simulink subsystem "SCIOutAbstractionOpenLoop"  (R2024b)
settings: Solver=VariableStepAuto  StartTime=0.0  StopTime=10.0  RelTol=1e-3
libraries: svdutilitieslib x1
settings Model: Creator=The MathWorks, Inc.  LastModifiedBy=snarayan
settings RTWCC: GPUComputeCapability=3.5  LargeConstantGeneration=WriteOnlyDNNConstantsToDataFiles

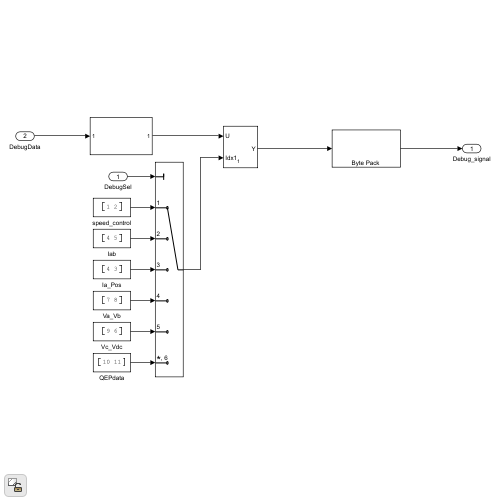
[thumbnail: Simulink's stored preview of the top-level diagram]
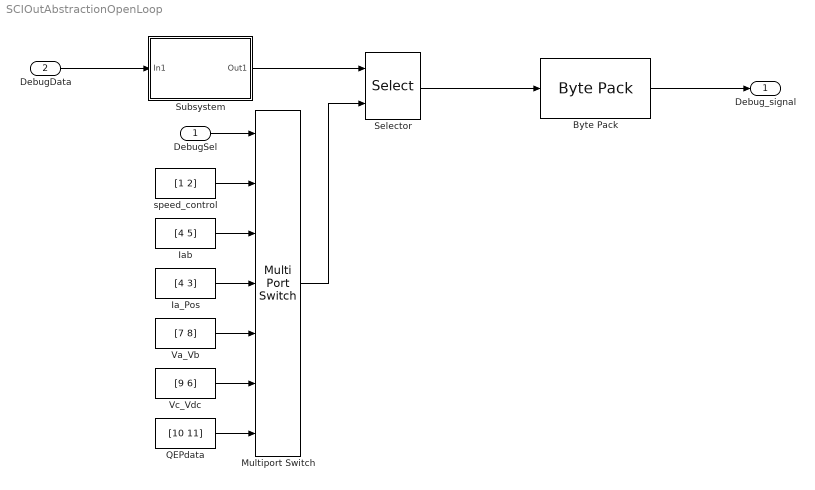
== system SCIOutAbstractionOpenLoop ==
  DebugSel : Inport
  DebugData : Inport  Port=2
  Byte Pack : svdutilitieslib/Byte Pack  maskPackedDataType=uint8  datatypes={'single'}  byteAlign=1  blockPlatform=tic2000
  Ia_Pos : Constant  Value=[4 3]  OutDataTypeStr=uint16  SampleTime=-1
  Iab : Constant  Value=[4 5]  OutDataTypeStr=uint16  SampleTime=-1
  Multiport Switch : MultiPortSwitch  Inputs=6  DiagnosticForDefault=Warning  OutDataTypeStr=uint16  RndMeth=Simplest  SaturateOnIntegerOverflow=off  InputSameDT=off
  QEPdata : Constant  Value=[10 11]  OutDataTypeStr=uint16  SampleTime=-1
  Selector : Selector  InputPortWidth=11  IndexOptions=Index vector (port)  Indices=[1 3]  OutputSizes=1
  Subsystem : Subsystem
  Va_Vb : Constant  Value=[7 8]  OutDataTypeStr=uint16  SampleTime=-1
  Vc_Vdc : Constant  Value=[9 6]  OutDataTypeStr=uint16  SampleTime=-1
  speed_control : Constant  Value=[1 2]  OutDataTypeStr=uint16  SampleTime=-1
  Debug_signal : Outport
  wires:
  speed_control/1 -> Multiport Switch/2
  Multiport Switch/1 -> Selector/2
  DebugSel/1 -> Multiport Switch/1
  Selector/1 -> Byte Pack/1
  Byte Pack/1 -> Debug_signal/1
  Iab/1 -> Multiport Switch/3
  Ia_Pos/1 -> Multiport Switch/4
  DebugData/1 -> Subsystem/1(In1)
  Subsystem/1(Out1) -> Selector/1
  QEPdata/1 -> Multiport Switch/7
  Vc_Vdc/1 -> Multiport Switch/6
  Va_Vb/1 -> Multiport Switch/5

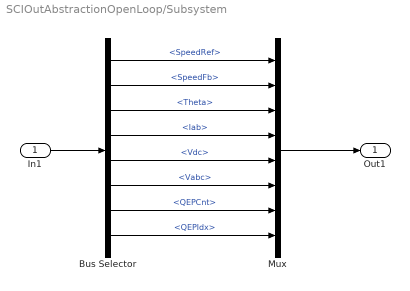
== system SCIOutAbstractionOpenLoop/Subsystem ==
  In1 : Inport
  Bus Selector : BusSelector  OutputSignals=SpeedRef,SpeedFb,Theta,Iab,Vdc,Vabc,QEPCnt,QEPIdx
  Mux : Mux  Inputs=8
  Out1 : Outport
  wires:
  Bus Selector/8 -> Mux/8  "<QEPIdx>"
  Bus Selector/7 -> Mux/7  "<QEPCnt>"
  Bus Selector/6 -> Mux/6  "<Vabc>"
  Bus Selector/5 -> Mux/5  "<Vdc>"
  Mux/1 -> Out1/1
  In1/1 -> Bus Selector/1
  Bus Selector/3 -> Mux/3  "<Theta>"
  Bus Selector/1 -> Mux/1  "<SpeedRef>"
  Bus Selector/4 -> Mux/4  "<Iab>"
  Bus Selector/2 -> Mux/2  "<SpeedFb>"
